simulink model "ADCS_r2017b_may8morning"  (R2017b)
settings: Solver=VariableStepAuto  StartTime=0.0  StopTime=10.0  RelTol=1e-3
undefined symbols (not defined in the file or in its folder): delta_t, SC, SS
libraries: sharedutil x3, vrlib x2
(part 2 of 2)

== matlab function ADCS_r2017b_may8morning/Satellite Simulator/Environment/Subsystem/MATLAB Function ==
  data: decYear input; B_ned output; yearLastEpoch input; lastgh input; ghslope input; latitude input; longitude input; altitude input
function B_ned  = igrf_mag_field(decYear, yearLastEpoch, lastgh, ghslope, latitude, longitude, altitude)
% IGRF Earth's magnetic field from IGRF model.
% 
% Usage: B = IGRF(COEFS, LATITUDE, LONGITUDE, ALTITUDE)
% 
% Calculates the components of the Earth's magnetic field using the
% International Geomagnetic Reference Field (IGRF) model. The inputs for
% the position can be scalars.
% 
% When all the coordinate inputs are scalars, the function can be run more
% efficiently by providing the proper IGRF coefficient vector for a given
% time rather than the time itself. This mode is useful when making
% multiple calls to the function while keeping the time the same (meaning
% the coefficients will be the same for each run) as loading the
% coefficients can be the most time-consuming part of the function. The
% coefficient vector can be easily loaded using the function LOADIGRFCOEFS.
% This mode is assumed when all the coordinate inputs are scalars and the
% first input is a vector. In this case, the coefficient vector should be
% formatted as (LOADIGRFCOEFS provides this):
% 
%   [g(n=1,m=0) g(n=1,m=1) h(n=1,m=1) g(n=2,m=0) g(n=2,m=1) h(n=2,m=1) ...]
% 
% Regardless of the size of the inputs, the outputs will be column vectors.
% If only one output is requested, B = [BX(:), BY(:), BZ(:)] is output.
% Note that the other parameters the IGRF gives can be computed from BX,
% BY, and BZ as:
% 
%   Horizonal intensity: hypot(BX, BY) (i.e., sqrt(BX.^2 + BY.^2) )
%   Total intensity: hypot(BX, hypot(BY, BZ))
%   Declination: atan2(BY, BX)
%   Inclination: atan(BZ./hypot(BX, BY))
% 
% This function relies on having the file igrfcoefs.mat in the MATLAB
% path to function properly when a time is input. If this file cannot be
% found, this function will try to create it by calling GETIGRFCOEFS.
% 
% The IGRF is a spherical harmonic expansion of the Earth's internal
% magnetic field. Currently, the IGRF model is valid between the years 1900
% and 2015. See the health warning for the IGRF model here:
% http://www.ngdc.noaa.gov/IAGA/vmod/igrfhw.html
% 
% Reference:
% International Association of Geomagnetism and Aeronomy, Working Group 
% V-MOD (2010), International Geomagnetic Reference Field: the eleventh
% generation, _Geophys. J. Int._, _183_(3), 1216-1230, 
% doi:10.1111/j.1365-246X.2010.04804.x.
% 
% Inputs:
%   -COEFS: Instead of inputting a time, you can simply specify the proper
%   coefficients for the time you want by inputting in the first argument
%   the proper coefficient vector from igrfcoefs.mat.
%   -LATITUDE: Geocentric or geodetic latitude in degrees.
%   -LONGITUDE: Geocentric or geodetic longitude in degrees.
%   -ALTITUDE: For geodetic coordiates, the height in km above the Earth's
%   surface. For geocentric coordiates, the radius in km from the center of
%   the Earth.

% 
% Outputs:
%   -BX: Northward component of the magnetic field in nanoteslas (nT).
%   -BY: Eastward component of the magnetic field in nT.
%   -BZ: Downward component of the magnetic field in nT.
%   -B: [BX(:), BY(:), BZ(:)].
% 
% See also: LOADIGRFCOEFS, GETIGRFCOEFS, IGRFLINE, DATENUM, IGRF11MAGM.


%%%%%%%%%%%%%%%%%%%%%%%%%%%%%%%%%%%%%%%%%%%%%%%%%%%%%%%%%%%%%%%%%%%%%%%%%%%
%%%%%%%%%%%%%%%%%%%        IGRF scalar function.        %%%%%%%%%%%%%%%%%%%
%%%%%%%%%%%%%%%%%%%%%%%%%%%%%%%%%%%%%%%%%%%%%%%%%%%%%%%%%%%%%%%%%%%%%%%%%%%
%function [Bx, By, Bz] = igrfs(time, latitude, longitude, altitude, coord)

% Fundamental constant.
Rearth_km = 6371.2;
altitude=altitude/1000;
%%% SPHERICAL COORDINATE CONVERSION %%%
% Convert the latitude, longitude, and altitude coordinates input into
% spherical coordinates r (radius), theta (inclination angle from +z axis),
% and phi (azimuth angle from +x axis).
% We want cos(theta) and sin(theta) rather than theta itself.
costheta = cos((90 - latitude)*pi/180);
sintheta = sin((90 - latitude)*pi/180);

% Convert from geodetic coordinates to geocentric coordinates if necessary.
% This method was adapted from igrf11syn, which was a conversion of the
% IGRF subroutine written in FORTRAN.

    a = 6378.137; f = 1/298.257223563; b = a*(1 - f);
    rho = hypot(a*sintheta, b*costheta);
    r = sqrt( altitude.^2 + 2*altitude.*rho + ...
        (a^4*sintheta.^2 + b^4*costheta.^2) ./ rho.^2 );
    cd = (altitude + rho) ./ r;
    sd = (a^2 - b^2) ./ rho .* costheta.*sintheta./r;
    oldcos = costheta;
    costheta = costheta.*cd - sintheta.*sd;
    sintheta = sintheta.*cd + oldcos.*sd;


% Convert longitude to radians.
phi = longitude*pi/180;

%%% GET PROPER IGRF COEFFICIENTS %%%

gh=lastgh+ghslope*(decYear-yearLastEpoch);
nmax = sqrt(numel(gh) + 1) - 1;


% We need cos(m*phi) and sin(m*phi) multiple times, so precalculate into a
% vector here:
cosphi = cos((1:nmax)*phi);
sinphi = sin((1:nmax)*phi);

Pmax = (nmax+1)*(nmax+2)/2;

%%% BEGIN MAGNETIC FIELD CALCULATION %%%
% Initialize variables used in for loop below.
Br = 0; Bt = 0; Bp = 0;
 P = zeros(1, Pmax);  P(1) = 1;  P(3) = sintheta;
dP = zeros(1, Pmax); dP(1) = 0; dP(3) = costheta;

% For this initial condition, the first if will result in n = 1, m = 0.
m = 1; n = 0; coefindex = 1;

a_r = (Rearth_km/r)^2;

% Increment through all the n's and m's. gh will be a vector with g
% followed by h for incrementing through n and m except when h would be
% redundant (i.e., when m = 0).
for Pindex = 2:Pmax
    
    % Increment to the next n when m becomes larger than n.
    if n < m
        m = 0;
        n = n + 1;
        a_r = a_r*(Rearth_km/r); % We need (Rearth_km./r)^(n+2)
    end
    
    % Calculate P and dP. They are given recursively according to:
    % 
    % P(0, 0) = 1, P(1, 1) = sin(theta) <- Specified above
    % P(n, n) = sqrt(1 - 1/(2n))*sin(theta)*P(n-1, n-1)
    % P(n, m) = (2n - 1)/sqrt(n^2 - m^2)*cos(theta)*P(n-1, m) -
    %     sqrt(((n-1)^2 - m^2) / (n^2 - m^2)) * P(n-2, m)
    % 
    % dP(0, 0) = 0, dP(1, 1) = cos(theta) <- Specified above
    % dP(n, n) = sqrt(1 - 1/(2n))*(sin(theta)*dP(n-1, n-1) +
    %     cos(theta)*P(n-1, n-1))
    % dP(n, m) = (2n - 1)/sqrt(n^2 - m^2)*(cos(theta)*dP(n-1, m) -
    %     sin(theta)*P(n-1, m)) - sqrt(((n-1)^2 - m^2)/(n^2 - m^2))*
    %     dP(n-2, m)
    if m < n && Pindex ~= 3 % (Pindex=3 is n=1, m=1, initial cond. above)
        last1n = Pindex - n;
        last2n = Pindex - 2*n + 1;
        P(Pindex) = (2*n - 1)/sqrt(n^2 - m^2)*costheta*P(last1n) - ...
            sqrt(((n-1)^2 - m^2) / (n^2 - m^2)) * P(last2n);
        dP(Pindex) = (2*n - 1)/sqrt(n^2 - m^2)*(costheta*dP(last1n) - ...
            sintheta*P(last1n)) - sqrt(((n-1)^2 - m^2) / (n^2 - m^2)) * ...
            dP(last2n);
    elseif Pindex ~= 3
        lastn = Pindex - n - 1;
        P(Pindex) = sqrt(1 - 1/(2*m))*sintheta*P(lastn);
        dP(Pindex) = sqrt(1 - 1/(2*m))*(sintheta*dP(lastn) + ...
            costheta*P(lastn));
    end
    
    % Calculate the magnetic field components as a running sum. Find
    % explicit expressions for these in Global Earth Physics: a Handbook of
    % Physical Constants by Thomas J. Aherns (1995), pg. 49. Link:
    % http://books.google.com/books?id=aqjU_NHyre4C&lpg=PP1&dq=Global%20
    % earth%20physics%3A%20a%20handbook%20of%20physical%20constants&pg=PA49
    % #v=onepage&q&f=false
    % (except equation 6 is missing a required 1/sin(theta) and m; correct
    % equations on page 5 (equations 3a-3c) of:
    % http://hanspeterschaub.info/Papers/UnderGradStudents/
    % MagneticField.pdf)
    if m == 0 % Implies h = 0, so only coefficient in gh is g
        coef = a_r*gh(coefindex); %*cos(0*phi) = 1
        Br = Br + (n+1)*coef*P(Pindex);
        Bt = Bt - coef*dP(Pindex);
        % Bp is 0 for m = 0.
        coefindex = coefindex + 1; % Only need to skip over g this time.
    else
        coef = a_r*(gh(coefindex)*cosphi(m) + gh(coefindex+1)*sinphi(m));
        Br = Br + (n+1)*coef*P(Pindex);
        Bt = Bt - coef*dP(Pindex);
        if sintheta == 0 % Use different formula when dividing by 0.
            Bp = Bp - costheta*a_r*(-gh(coefindex)*sinphi(m) + ...
                gh(coefindex+1)*cosphi(m))*dP(Pindex);
        else
            Bp = Bp - 1/sintheta*a_r*m*(-gh(coefindex)*sinphi(m) + ...
                gh(coefindex+1)*cosphi(m))*P(Pindex);
        end
        coefindex = coefindex + 2; % Skip over g and h this time.
    end
    
    % Increment m.
    m = m + 1;
    
end

% Convert from spherical to (x,y,z) = (North,East,Down).
Bx = -Bt;
By = Bp;
Bz = -Br;

% Convert back to geodetic coordinates if necessary.
Bx_old = Bx;
Bx = Bx.*cd + Bz.*sd;
Bz = Bz.*cd - Bx_old.*sd;

B_ned = [Bx;By;Bz];

== matlab function ADCS_r2017b_may8morning/Satellite Simulator/Kinematics/Calc Coordinate Transforms/MATLAB Function ==
  data: lati input; R_ecef2ned output; long input
function R_ecef2ned   = calc_ECEF_to_NED( lati, long )
%Given the latitude and longitude, returns the rotation matrix to tranform
%ECEF coordinates into NED coordinates.
%   Detailed explanation goes here
phi = lati*pi/180; %radians
lam = long*pi/180; %radians
sinp = sin(phi);
sinl = sin(lam);
cosp = cos(phi);
cosl = cos(lam);

A = zeros(3,3);
A(1,1) = -1*sinp*cosl;
A(1,2) = -1*sinp*sinl;
A(1,3) =    cosp;
A(2,1) = -1*sinl;
A(2,2) =    cosl;
A(2,3) = 0;
A(3,1) = -1*cosp*cosl;
A(3,2) = -1*cosp*sinl;
A(3,3) = -1*sinp;

R_ecef2ned = A;
end

== matlab function ADCS_r2017b_may8morning/Satellite Simulator/Kinematics/Calc Coordinate Transforms/Calc_R_eci2mci ==
  data: JD_i input; R_eci2mci output
function R_eci2mci = fcn(JD_i)
R_eci2mci = [1,0,0;
             0,1,0;
             0,0,1];
end

== matlab function ADCS_r2017b_may8morning/Satellite Simulator/External Forces and Torques/External Torques/Grav gradient earth/MATLAB Function ==
  data: rIr input; tor output; r_eci input; GM input
function tor = fcn(rIr, r_eci, GM)
r = norm(r_eci);
tor = (3*GM)/(r^3) * rIr;
end

== matlab function ADCS_r2017b_may8morning/Satellite Simulator/External Forces and Torques/External Torques/Grav gradient moon/MATLAB Function ==
  data: rIr input; tor output; r_mci input; GM input
function tor = fcn(rIr, r_mci, GM)
r = norm(r_mci);
tor = (3*GM)/(r^3) * rIr;

== matlab function ADCS_r2017b_may8morning/Satellite Simulator/Actuators/RCS Model ==
  data: command input; force_body output; torque_body output; moment_arms input; norm_dir input; max_thrust input
function [force_body, torque_body] = fcn(command, moment_arms, norm_dir, max_thrust)
%input: 12 commands, on range from 0-1, corresponding to which thruster to fir
 force_body = [0;0;0];
torque_body = [0;0;0];
num = length(command); %number of thrusters
for i=1:num
     force_body =  force_body + max_thrust*command(i)*norm_dir(:,i);
    torque_body = torque_body + max_thrust*command(i)*moment_arms(:,i);
end

== matlab function ADCS_r2017b_may8morning/Satellite Simulator/Environment/Earth State in HCI ==
  data: planet_id input; rHCI output; jd input; vHCI output
function [rHCI, vHCI] = AA279planet_state(planet_id, jd)
% Returns heliocentric position and velocity of planet at given time
%
% AA279 Function Library
% Last modified: 22 April 2016 by Andrew K. Barrows

% Physical constants from http://ssd.jpl.nasa.gov/horizons.cgi  Feb 2014
km_per_au = 149597870.700; % [km/AU]
musun     = 1.3271244004193938e11; % [km^3/sec^2]

% Get data for selected planet
[j2000_elements, rates] = AA279j2000_planetary_elements(planet_id);

% Find elements at given time
elements = j2000_elements + rates*(jd - 2451545)/36525;

a = elements(1)*km_per_au; % semi-major axis
ecc = elements(2); % eccentricity

p = a*(1 - ecc*ecc); % [km]

inc = elements(3); % [deg] inclination (assume stays in [-90 +90] range)

LAN = elements(4); % [deg] longitude of ascending node
while LAN >= 360.0
    LAN = LAN - 360.0; 
end
while LAN < 0.0
    LAN = LAN + 360.0;
end

omega_bar = elements(5); % [deg] longitude of perihelion
while omega_bar >= 360.0
    omega_bar = omega_bar - 360.0; 
end
while omega_bar < 0.0
    omega_bar = omega_bar + 360.0;
end

L = elements(6); % [deg] mean longitude
while L >= 360.0
    L = L - 360.0; 
end
while L < 0.0
    L = L + 360.0;
end  

omega = omega_bar - LAN; % [deg] argument of perihelion
while omega >= 360.0
    omega = omega - 360.0; 
end
while omega < 0.0
    omega = omega + 360.0;
end 

M = L - omega_bar; % [deg] mean anomaly
while M >= 360.0
    M = M - 360.0; 
end
while M < 0.0
    M = M + 360.0;
end 

% Find eccentric anomaly by solving Kepler's equation
E = AA279solve_kepler(M*pi/180, ecc, 1e-10); % [rad]

% Find position and velocity of planet in perifocal coordinates
sinnu = (sin(E)*sqrt(1.0-ecc*ecc))/(1.0-ecc*cos(E));
cosnu = (cos(E)-ecc)/(1.0-ecc*cos(E));
r = p/(1.0+ecc*cosnu); % Trajectory Equation
O_r_P__peri = [r*cosnu; r*sinnu; 0.0];
sqrtmuoverp = sqrt(musun/p);
peri_v_P__peri = [-sqrtmuoverp*sinnu; sqrtmuoverp*(ecc+cosnu); 0.0];
      
% Convert perifocal coordinates to heliocentric coordinates
sinLAN = sin(LAN*pi/180.0);
cosLAN = cos(LAN*pi/180.0);
sininc = sin(inc*pi/180.0);
cosinc = cos(inc*pi/180.0);
sinomega = sin(omega*pi/180.0);
cosomega = cos(omega*pi/180.0);
heli_C_peri = [+cosLAN*cosomega-sinLAN*sinomega*cosinc ...
                  -cosLAN*sinomega-sinLAN*cosomega*cosinc ...
                      +sinLAN*sininc; ...
              +sinLAN*cosomega+cosLAN*sinomega*cosinc ...
                  -sinLAN*sinomega+cosLAN*cosomega*cosinc ...
                      -cosLAN*sininc; ...       
              +sinomega*sininc ...
                  +cosomega*sininc ...
                      +cosinc];
rHCI = heli_C_peri*O_r_P__peri;
vHCI = heli_C_peri*peri_v_P__peri; % because heli_omega_peri = 0

end % terminates MATLAB function


function [E] = AA279solve_kepler(M, e, tol)
% Solves Kepler's Equation using Newton's method
%
% AA279 Function Library
% Last modified: 22 April 2016 by Andrew K. Barrows
%
% E    Eccentric Anomaly [rad]
% M    Mean Anomaly [rad]
% e    eccentricity [dimensionless]
% tol  tolerance value on E for stopping iteration [rad]

E   = (pi+M)/2;  % initial guess
err = tol + 1.0; % ensures at least one iteration will take place

% Iterate using Newton's method
while err >= tol
    Enew = E + (M-E+e*sin(E))/(1-e*cos(E));
    err = abs(Enew-E);
    E = Enew;
end

end % terminates MATLAB function

function [elements, rates] = AA279j2000_planetary_elements(planet_id)
% Returns a planet's J2000 orbital elements and centennial rates
%
% AA279 Function Library
% Last modified: 22 April 2016 by Andrew K. Barrows
%
% Adapted from Orbital Mechanics for Engineering Students by Howard Curtis
% 
% Data valid for the period 1800 AD - 2050 AD
% Source of data: http://ssd.jpl.nasa.gov/?planet_pos
%
% planet_id: 1 through 9, for Mercury through Pluto
%  
% elements:  row vector of J2000 orbital elements for "planet_id"
%                a             semimajor axis [AU]
%                e             eccentricity
%                i             inclination [deg]
%                OMEGA         longitude of the ascending node [deg]
%                omega_bar     longitude of perihelion [deg]
%                L             mean longitude [deg]                   
%                                         
% rates:     row vector of J2000 centennial rates for "planet_id"    
%                a_dot         [AU/cty] (AU per century)
%                e_dot         [1/cty]
%                i_dot         [deg/cty]
%                OMEGA_dot     [deg/cty]
%                omega_bar_dot [deg/cty]
%                L_dot         [deg/cty]
%
%     a           e          i          OMEGA      omega_bar        L

J2000_elements = ...
[0.38709927  0.20563593  7.00497902  48.33076593  77.45779628  252.25032350
 0.72333566  0.00677672  3.39467605  76.67984255 131.60246718  181.97909950 
 1.00000261  0.01671123 -0.00001531   0.0        102.93768193  100.46457166 
 1.52371034  0.09339410  1.84969142  49.55953891 -23.94362959 	-4.55343205
 5.20288700  0.04838624  1.30439695 100.47390909  14.72847983 	34.39644501
 9.53667594  0.05386179  2.48599187 113.66242448  92.59887831 	49.95424423
19.18916464  0.04725744  0.77263783  74.01692503 170.95427630  313.23810451
30.06992276  0.00859048  1.77004347 131.78422574  44.96476227  -55.12002969 
39.48211675  0.24882730 17.14001206 110.30393684 224.06891629  238.92903833];

centennial_rates = ... 
[0.00000037  0.00001906 -0.00594749 -0.12534081  0.16047689  149472.67411175 
 0.00000390 -0.00004107 -0.00078890 -0.27769418  0.00268329	  58517.81538729  
 0.00000562 -0.00004392 -0.01294668  0.0         0.32327364   35999.37244981  
 0.0001847 	 0.00007882 -0.00813131 -0.29257343  0.44441088   19140.30268499  
-0.00011607 -0.00013253 -0.00183714  0.20469106	 0.21252668    3034.74612775 
-0.00125060 -0.00050991  0.00193609 -0.28867794 -0.41897216    1222.49362201
-0.00196176 -0.00004397 -0.00242939  0.04240589  0.40805281 	428.48202785 
 0.00026291  0.00005105  0.00035372 -0.00508664 -0.32241464 	218.45945325 
-0.00031596  0.00005170  0.00004818 -0.01183482 -0.04062942 	145.20780515]; 
 
elements = J2000_elements(planet_id, :);
rates = centennial_rates(planet_id, :);
end % terminates MATLAB function

== matlab function ADCS_r2017b_may8morning/Satellite Simulator/Environment/Moon State in ECI ==
  data: time input; moon_eci output
function moon_eci = fcn(time)

moon_eci = [0;0;0];
end

== matlab function ADCS_r2017b_may8morning/Satellite Simulator/Environment/calc_eclipse ==
  data: sun_eci input; eclipse output; moon_eci input; r_eci input
function eclipse = fcn(sun_eci, moon_eci, r_eci)

eclipse_earth = 0;
eclipse_moon  = 0;
sun_mci = sun_eci - moon_eci;
  r_mci =   r_eci - moon_eci;

%check for ecclipse with earth
%ref: Vallado, page 201
R_e = 6378137;
f = 1/298.257223563;
e = sqrt(2*f-f*f);
d_sun = norm(sun_eci);
d_sat = norm(r_eci);
temp = 1/sqrt(1-e^2);
sun_eci(3) = sun_eci(3)*temp;
  r_eci(3) =   r_eci(3)*temp;
if (abs(d_sun^2 + d_sat^2 - 2*dot(sun_eci,r_eci)) < 0.0001)
    t_min = 0;
else
    t_min = (d_sun^2 - dot(sun_eci,r_eci)) / (d_sun^2+d_sat^2-2*dot(sun_eci,r_eci));
end

if ( t_min < 0 || t_min > 1)
    eclipse_earth = 1;
else
    distsqrd = ((1-t_min)*d_sun^2+t_min*dot(sun_eci,r_eci))/(R_e^2);
    if distsqrd > 1
        eclipse_earth = 1;
    else
        eclipse_earth = 0;
    end
end

%check for eclipse with moon
R_m = 1738100;
f = 0.0012;
e = sqrt(2*f-f*f);
d_sun = norm(sun_mci);
d_sat = norm(r_mci);
temp = 1/sqrt(1-e^2);
sun_mci(3) = sun_mci(3)*temp;
  r_mci(3) =   r_mci(3)*temp;
if (abs(d_sun^2 + d_sat^2 - 2*dot(sun_mci,r_mci)) < 0.0001)
    t_min = 0;
else
    t_min = (d_sun^2 - dot(sun_mci,r_mci)) / (d_sun^2+d_sat^2-2*dot(sun_mci,r_mci));
end

if ( t_min < 0 || t_min > 1)
    eclipse_moon = 1;
else
    distsqrd = ((1-t_min)*d_sun^2+t_min*dot(sun_mci,r_mci))/(R_m^2);
    if distsqrd > 1
        eclipse_moon = 1;
    else
        eclipse_moon = 0;
    end
end


if(eclipse_earth || eclipse_moon)
    eclipse = 1;
else
    eclipse = 0;
end

end

== matlab function ADCS_r2017b_may8morning/Satellite Simulator/External Forces and Torques/External Forces/Aero Drag ==
  data: r_eci input; a_body output; v_eci input; R_eci2body input; CD input
function a_body = fcn(r_eci, v_eci, R_eci2body, CD)

a_body = [0;0;0];
end

== matlab function ADCS_r2017b_may8morning/Satellite Simulator/External Forces and Torques/External Forces/Earth Gravity ==
  data: r_eci input; a_eci output; GM_Earth input
function a_eci = accelPointMass(r_eci, GM_Earth)
a_eci = -GM_Earth*r_eci./norm(r_eci)^3;
end

== matlab function ADCS_r2017b_may8morning/Satellite Simulator/External Forces and Torques/External Forces/Moon Gravity ==
  data: r_eci input; a_eci output; moon_eci input; GM_Moon input
function a_eci = accelPointMass(r_eci, moon_eci, GM_Moon)
r_eci = r_eci - moon_eci;
a_eci = -GM_Moon*r_eci./norm(r_eci)^3;
end

== matlab function ADCS_r2017b_may8morning/Satellite Simulator/External Forces and Torques/External Forces/Solar Radiation Pressure ==
  data: r_eci input; a_body output; sun_eci input; R_eci2body input; eclipse input; unitPtVec input; area_per_face input; mass input
function a_body = srp(r_eci, sun_eci, R_eci2body, eclipse, unitPtVec, area_per_face,mass)
sat2sun_eci = sun_eci - r_eci;
sat2sun_eci_unit = sat2sun_eci / norm(sat2sun_eci);
solar_flux = 1361 * (149598023000^2)/(norm(sat2sun_eci)^2); %W/m2
sun_dir_body = R_eci2body * sat2sun_eci_unit;
num_faces = length(area_per_face); %should be 6
c = 299792458; %m/s

F = [0;0;0];
for i=1:num_faces
    projected_area = area_per_face(i) * dot(unitPtVec(:,i), sun_dir_body);
    if(projected_area < 0)  %face is not facing sun
        projected_area = 0;
    end
    P = solar_flux/c; %N/m2 
    F = F+P*projected_area;
end

if eclipse
    a_body = [0;0;0];
else
    a_body = (1/mass)*F;
end

== matlab function ADCS_r2017b_may8morning/Satellite Simulator/External Forces and Torques/External Forces/Sun Gravity ==
  data: r_eci input; a_eci output; sun_eci input; GM_sun input
function a_eci = accelPointMass(r_eci, sun_eci, GM_sun)
r_eci = r_eci - sun_eci;
a_eci = -GM_sun*r_eci./norm(r_eci)^3;
end

== matlab function ADCS_r2017b_may8morning/Satellite Simulator/External Forces and Torques/External Torques/Aero Torque ==
  data: f_aero_body input; tor output; moment_arms input
function tor = fcn(f_aero_body, moment_arms)
tor = [0;0;0];
for i=length(f_aero_body(1,:))
    tor = tor + Skew(moment_arms(:,i))*f_aero_body(:,i);
end
end

function S = Skew(v)

S =[0 -v(3) v(2)
v(3) 0 -v(1)
-v(2) v(1) 0];
end

== matlab function ADCS_r2017b_may8morning/Satellite Simulator/External Forces and Torques/External Torques/SRP Torque ==
  data: f_SRP_body input; tor output; moment_arms input
function tor = fcn(f_SRP_body, moment_arms)
tor = [0;0;0];
for i=length(f_SRP_body(1,:))
    tor = tor + Skew(moment_arms(:,i))*f_SRP_body(:,i);
end
end

function S = Skew(v)

S =[0 -v(3) v(2)
v(3) 0 -v(1)
-v(2) v(1) 0];
end

== matlab function ADCS_r2017b_may8morning/Satellite Simulator/Kinematics/Rotation Kinematics/Euler Equations ==
  data: w input; w_dot output; tor input; I input
function w_dot = fcn(w, tor, I)

w_dot = -I\(Skew(w)*I*w-tor);

% w_dot = zeros(size(w));
% wx = w(1); wy = w(2); wz = w(3);
% Ix = I(1,1); Iy = I(2,2); Iz = I(3,3);
% w_dot(1) = (tor(1) - (Iz-Iy)*wx*wz)/Ix;  %update this to work in body axis
% w_dot(2) = (tor(2) - (Ix-Iz)*wz*wx)/Iy;
% w_dot(3) = (tor(3) - (Iy-Ix)*wx*wy)/Iz;
end


function S = Skew(v)
S = [0 -v(3) v(2)
    v(3) 0 -v(1)
    -v(2) v(1) 0];
end

== matlab function ADCS_r2017b_may8morning/Satellite Simulator/Sensors/Sun sensor model ==
  data: r_eci input; sun_eci input; sun_meas output; R_eci2body input; noise input; eclipse input; unitPtVec input
function sun_meas = fcn(r_eci, sun_eci, R_eci2body, noise, eclipse, unitPtVec)
sat2sun_eci = sun_eci - r_eci;
sat2sun_eci_unit = sat2sun_eci / norm(sat2sun_eci);
solar_flux = 1361 * (149598023000^2)/(norm(sat2sun_eci)^2); %W/m2
sun_dir_body = R_eci2body * sat2sun_eci_unit;
num_faces = length(unitPtVec); %should be 6

sun_meas = zeros(num_faces, 1);
for i=1:num_faces
    P = solar_flux * dot(unitPtVec(:,i), sun_dir_body);
    if(P < 0 || eclipse) %face is wrong direction
        P = 0;
    end
    %add moon albido
    %%%P = P + fxn(moon_position, orientation)
    P = P/1361;
    sun_meas(i) = P; 
end

sun_meas = sun_meas + noise*randn([6,1]);

== matlab function ADCS_r2017b_may8morning/Satellite Simulator/Sensors/Star tracker model ==
  data: q_actual input; w_body input; q_meas output; noise input; w_limit input
function q_meas = fcn(q_actual, w_body, noise, w_limit)

if norm(w_body) < w_limit
    q_meas = [0;0;0;0];
else
    q_meas = q_actual + noise*randn(4,1);
    q_meas = q_meas/norm(q_meas);
end

== matlab function ADCS_r2017b_may8morning/Satellite Simulator/Time Model/Date2JD ==
  data: date input; JD output
function JD = fcn(date)
year   = date(1);
month  = date(2);
day    = date(3);
hour   = date(4);
minute = date(5);
second = date(6);

% Calendar Date to Modified Julian Date
% From Montenbruck, Appendix A, page 321

% adjust for leap years
if month <=2
    y = year - 1;
    m = month + 12;
else
    y = year;
    m = month;
end

% leap days -- ASSUMPTION: we are beyond 4 Oct. 1582
B = y/400 - y/100 + y/4;

D = day + hour/24 + minute/(24*60) + second/(24*60*60);

MJD = 365*y - 679004 + B + (30.6001*(m+1)) + D;
JD = MJD + 2400000.5;
end


% %replace this with real function, find text book reference from 279a
% JD_Jan0_2020 = 2458848.5000;
% JD = JD_Jan0_2020 + (year-2020)*365 + month*30 + day + hour/24 + minute/(24*60) + second/(24*60*60);
